simulink model "celsiusConverter_KellenHassel"  (R2025b)
settings: Solver=VariableStepAuto  StartTime=0.0  StopTime=10.0  RelTol=1e-3

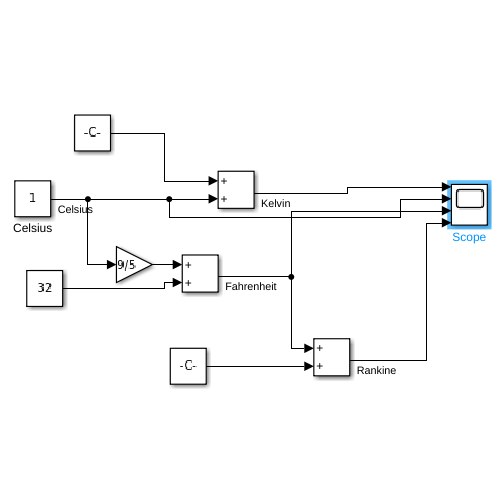
[thumbnail: Simulink's stored preview of the top-level diagram]
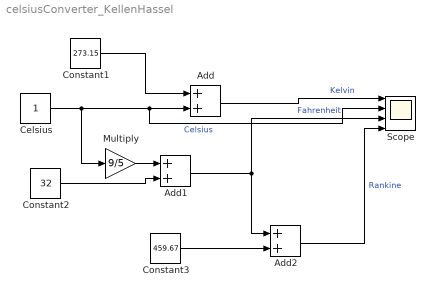
== system celsiusConverter_KellenHassel ==
  Add : Sum
  Add1 : Sum
  Add2 : Sum
  Celsius : Constant
  Constant1 : Constant  Value=273.15
  Constant2 : Constant  Value=32
  Constant3 : Constant  Value=459.67
  Multiply : Gain  Gain=9/5
  Scope : Scope  NumInputPorts=4
      settings: ActiveDisplayYMinimum=-125.24009518207885  ActiveDisplayYMaximum=619.60393890264572  YLabel=Temperature (°)
  wires:
  Celsius/1 -> Multiply/1, Scope/2, Add/2  "Celsius"
  Constant1/1 -> Add/1
  Add/1 -> Scope/1  "Kelvin"
  Multiply/1 -> Add1/1
  Constant2/1 -> Add1/2
  Add1/1 -> Add2/1, Scope/3  "Fahrenheit"
  Add2/1 -> Scope/4  "Rankine"
  Constant3/1 -> Add2/2
